simulink model "hw1_zoh2"  (R2017a)
settings: Solver=ode45  StartTime=0.0  StopTime=60.0  MaxStep=0.05  RelTol=1e-3  EnableMultiTasking=on
model workspace: external: MAT-File hw1_workspace.mat (data not in the file)
settings Model: Creator=antonio  LastModifiedBy=cleamoon
settings DataIOCC: LimitDataPoints=on  SaveFormat=Array
settings OptimizationCC: LifeSpan=inf
settings DebuggingCC: AllowSymbolicDim=off  SFUnexpectedBacktrackingDiag=warning  SFNoUnconditionalDefaultTransitionDiag=warning  SFExecutionAtInitializationDiag=none
settings HardwareCC: ProdBitPerPointer=32  ProdBitPerSizeT=32  ProdBitPerPtrDiffT=32  ProdLargestAtomicFloat=None  ProdIntDivRoundTo=Undefined  ProdEndianess=Unspecified  ProdWordSize=32  ProdHWDeviceType=32-bit Generic
settings ModelReferenceCC: PropagateSignalLabelsOutOfModel=off
settings GRTTargetCC: TargetLangStandard=C89/C90 (ANSI)  GeneratePreprocessorConditionals=Disable all
settings ConfigComp: CovMetricSettings=dw  CovHtmlReporting=on  CovSaveCumulativeToWorkspaceVar=on  CovSaveSingleToWorkspaceVar=on  CovExternalEMLEnable=off

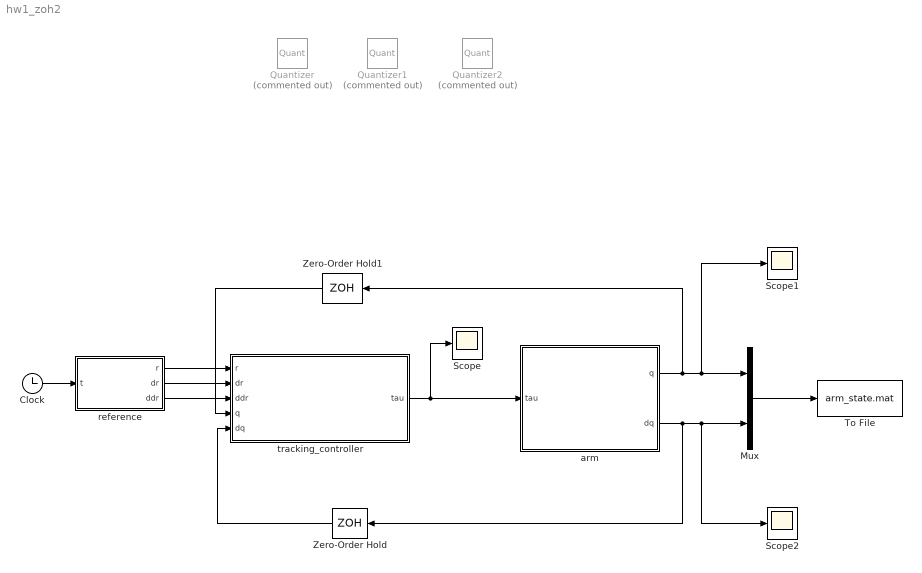
== system hw1_zoh2 ==
  Clock : Clock
  Mux : Mux  Inputs=2
  Quantizer : Quantizer  Commented=on  QuantizationInterval=5
  Quantizer1 : Quantizer  Commented=on  QuantizationInterval=5
  Quantizer2 : Quantizer  Commented=on  QuantizationInterval=5
  Scope : Scope
  Scope1 : Scope
  Scope2 : Scope
  To File : ToFile  Filename=arm_state.mat  MatrixName=x  SaveFormat=Timeseries
  Zero-Order Hold : ZeroOrderHold  SampleTime=0.30
  Zero-Order Hold1 : ZeroOrderHold  SampleTime=0.30
  arm : Subsystem
  reference : MATLAB Function  TreatAsAtomicUnit=on
  tracking_controller : MATLAB Function  TreatAsAtomicUnit=on
  wires:
  reference/1(r) -> tracking_controller/1(r)
  reference/2(dr) -> tracking_controller/2(dr)
  reference/3(ddr) -> tracking_controller/3(ddr)
  Clock/1 -> reference/1(t)
  Mux/1 -> To File/1
  arm/1(q) -> Zero-Order Hold1/1, Scope1/1, Mux/1
  arm/2(dq) -> Zero-Order Hold/1, Scope2/1, Mux/2
  tracking_controller/1(tau) -> arm/1(tau), Scope/1
  Zero-Order Hold1/1 -> tracking_controller/4(q)
  Zero-Order Hold/1 -> tracking_controller/5(dq)

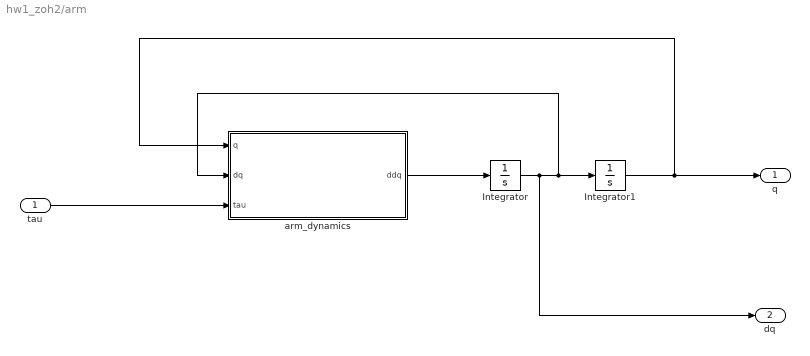
== system hw1_zoh2/arm ==
  tau : Inport
  Integrator : Integrator  InitialCondition=[0;0]
  Integrator1 : Integrator  InitialCondition=[0;0]
  arm_dynamics : MATLAB Function  TreatAsAtomicUnit=on
  q : Outport
  dq : Outport  Port=2
  wires:
  arm_dynamics/1(ddq) -> Integrator/1
  tau/1 -> arm_dynamics/3(tau)
  Integrator1/1 -> q/1, arm_dynamics/1(q)
  Integrator/1 -> dq/1, arm_dynamics/2(dq), Integrator1/1

== matlab function hw1_zoh2/arm/arm_dynamics ==
  data: q input; ddq output; dq input; tau input; I_1 data_store_memory; I_2 data_store_memory; m_1 data_store_memory; m_2 data_store_memory; l_1 data_store_memory; l_2 data_store_memory; g data_store_memory
function ddq = arm_dynamics(q, dq, tau)

coder.allowpcode('plain');
ddq = arm_dynamics_function(q, dq, tau);

end

== matlab function hw1_zoh2/tracking_controller ==
  data: r input; dr input; ddr input; q input; dq input; tau output; I_1 data_store_memory; I_2 data_store_memory; m_1 data_store_memory; m_2 data_store_memory; l_1 data_store_memory; l_2 data_store_memory; g data_store_memory
function tau = tracking_controller(r, dr, ddr, q, dq)


global m_1 m_2
global l_1 l_2
global I_1 I_2
global g

l_c1 = l_1/2;
l_c2 = l_2/2;

q1 = q(1);
q2 = q(2);

dq1 = dq(1);
dq2 = dq(2);

cq1 = cos(q1);
sq1 = sin(q1);

cq2 = cos(q(2));
sq2 = sin(q(2));

cq12 = cos(q(1)+q(2));


% Your code here

% Compute B
B_11 = m_1*l_c1^2 + I_1 + m_2*l_1^2 + m_2*l_c2^2 + 2*m_2*l_1*l_c2*cos(q2) + I_2;
B_12 = m_2*l_c2^2 + I_2 + m_1*l_1*l_c2*cos(q2);
B_21 = m_2*l_c2^2 + I_2 + m_1*l_1*l_c2*cos(q2);
B_22 = m_2*l_c2^2 + I_2;

B = [B_11, B_12; B_21, B_22];

% Compute N
N_11 = -m_2*l_1*l_c1*sin(q2)*dq2;
N_12 = -m_1*l_1*l_c1*sin(q2)*(dq1+dq2);
N_21 = m_1*l_c1^2*sin(q2)*dq1;
N_22 = 0;

N = [N_11, N_12; N_21, N_22];

% Compute pg
pg1 = m_1*g*l_c1*cos(q1) + m_2*g*l_1*cos(q1) + m_2*g*l_c2*cos(q1+q2);
pg2 = m_2*g*l_c2*cos(q1+q2);

pg = [pg1; pg2];

% Compute e and de
e = q-r;
de = dq-dr;

% Compute tau. Note that tau will be different for questions 4 and 7.
vdes = dr - e;
dvdes = ddr - de;
ev = dq - vdes;
tau = B*dvdes + N*vdes + pg - 3*dq - 3*ev;

%default
% tau = [0;0];

end

== matlab function hw1_zoh2/reference ==
  data: t input; r output; dr output; ddr output
function [r, dr, ddr] = reference(t)
% Assigns the reference as a function of time.
% The reference is assigned as
%  positions, velocities and accelerations
%  of the two joints. 

r = [pi/2; pi/4*sin(0.5*t)];
dr = [0; 0.5*pi/4*cos(0.5*t)];
ddr = [0; -0.5^2*pi/4*sin(0.5*t)];

% r = [pi/2; 0];
% dr = [0; 0];
% ddr = [0; 0];
